simulink model "AMR_VehicleSpeedReadout_24a"  (R2024a)
settings: configuration reference "SharedConfig" (kept outside this file)
undefined symbols (not defined in the file): gearbox_ratio, vehicle_track, vehicle_wheelbase, wheel_diameter
settings Model: DataDictionary=configuration_dictionary.sldd  Creator=matlab.cut  LastModifiedBy=matlab.cut
settings ConfigSetRef: SourceName=SharedConfig

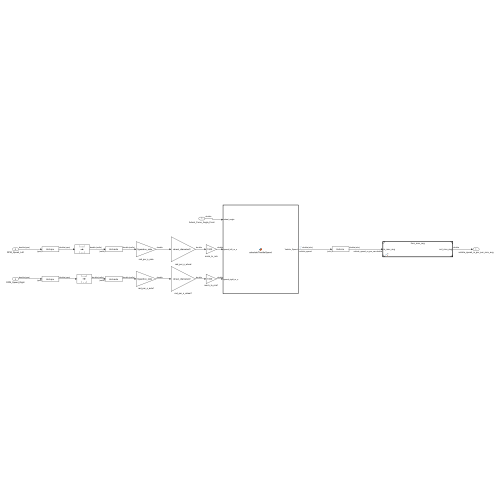
[thumbnail: Simulink's stored preview of the top-level diagram]
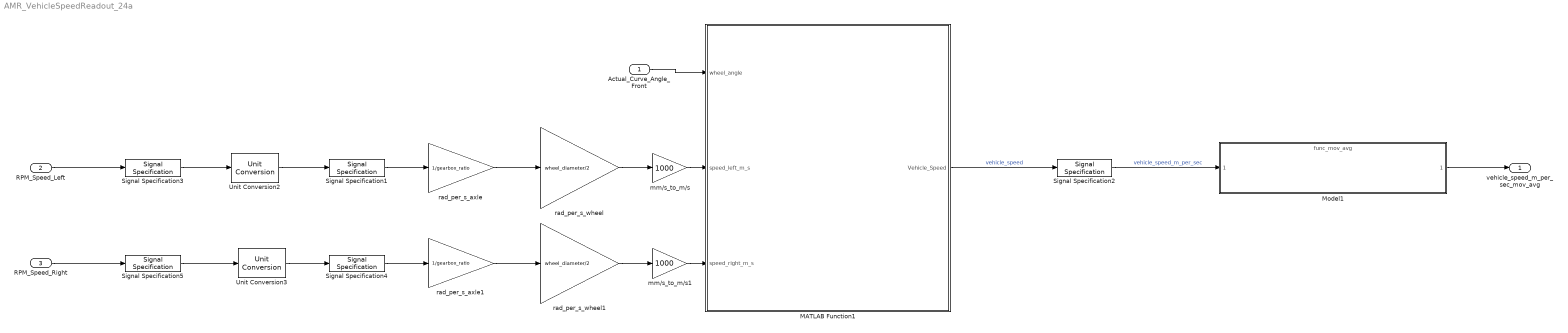
== system AMR_VehicleSpeedReadout_24a ==
  Actual_Curve_Angle_Front : Inport
  RPM_Speed_Left : Inport  Port=2
  RPM_Speed_Right : Inport  Port=3
  MATLAB Function1 : MATLAB Function  TreatAsAtomicUnit=on
  Model1 : ModelReference  ModelNameDialog=func_mov_avg.slx  SimulationMode=Normal  ModelReferenceVersion=2.6
  Signal Specification1 : SignalSpecification  Unit=rad/s
  Signal Specification2 : SignalSpecification  Unit=m/s
  Signal Specification3 : SignalSpecification  Unit=rpm
  Signal Specification4 : SignalSpecification  Unit=rad/s
  Signal Specification5 : SignalSpecification  Unit=rpm
  Unit Conversion2 : UnitConversion
  Unit Conversion3 : UnitConversion
  mm/s_to_m/s : Gain  Gain=1000
  mm/s_to_m/s1 : Gain  Gain=1000
  rad_per_s_axle : Gain  Gain=1/gearbox_ratio
  rad_per_s_axle1 : Gain  Gain=1/gearbox_ratio
  rad_per_s_wheel : Gain  Gain=wheel_diameter/2
  rad_per_s_wheel1 : Gain  Gain=wheel_diameter/2
  vehicle_speed_m_per_sec_mov_avg : Outport
  wires:
  MATLAB Function1/1(Vehicle_Speed) -> Signal Specification2/1  "vehicle_speed"
  Actual_Curve_Angle_Front/1 -> MATLAB Function1/1(wheel_angle)
  Signal Specification2/1 -> Model1/1  "vehicle_speed_m_per_sec"
  Model1/1 -> vehicle_speed_m_per_sec_mov_avg/1
  rad_per_s_axle/1 -> rad_per_s_wheel/1
  Signal Specification3/1 -> Unit Conversion2/1
  Unit Conversion2/1 -> Signal Specification1/1
  RPM_Speed_Left/1 -> Signal Specification3/1
  Signal Specification1/1 -> rad_per_s_axle/1
  rad_per_s_wheel/1 -> mm/s_to_m/s/1
  Unit Conversion3/1 -> Signal Specification4/1
  Signal Specification5/1 -> Unit Conversion3/1
  Signal Specification4/1 -> rad_per_s_axle1/1
  rad_per_s_axle1/1 -> rad_per_s_wheel1/1
  RPM_Speed_Right/1 -> Signal Specification5/1
  rad_per_s_wheel1/1 -> mm/s_to_m/s1/1
  mm/s_to_m/s/1 -> MATLAB Function1/2(speed_left_m_s)
  mm/s_to_m/s1/1 -> MATLAB Function1/3(speed_right_m_s)

== matlab function AMR_VehicleSpeedReadout_24a/MATLAB Function1 ==
  data: wheel_angle input; Vehicle_Speed output; speed_left_m_s input; speed_right_m_s input; vehicle_wheelbase parameter; vehicle_track parameter
function Vehicle_Speed = calculateThrottleSpeed(wheel_angle, speed_left_m_s, speed_right_m_s, vehicle_wheelbase, vehicle_track)


    % Navigation point rotantion radius:
    rotation_radius_nv = vehicle_wheelbase * tand(90 - abs(wheel_angle));

    % Steering wheel rotantion radius:
    rotation_radius_sw = vehicle_wheelbase * sqrt(tand(90 - abs(wheel_angle))^2 + 1 );


    vehicle_speed_from_left =  speed_left_m_s * rotation_radius_sw / (rotation_radius_nv - vehicle_track/2);
    vehicle_speed_from_right =  speed_right_m_s * rotation_radius_sw / (rotation_radius_nv + vehicle_track/2);
    
    Vehicle_Speed = mean([vehicle_speed_from_left, vehicle_speed_from_right]);

end
